simulink model "simulinkTVModel"  (R2023a)
settings: Solver=ode4  StartTime=0.0  StopTime=10.0  FixedStep=0.001  RelTol=1e-3
values from neighbouring files (symbols this model uses):
  K_att1 = lqr(AA,BA,QA,RA)    [TV_SIM_woCA.m]    (also in controllerParams.m)
  K_att2 = inv(BA'*BA)*BA'*AA    [controllerParams.m]
  K_pos1 = lqr(AP,BP,QP,RP)    [TV_SIM_woCA.m]    (also in controllerParams.m)
  K_pos2 = inv(BP'*BP)*BP'*AP    [controllerParams.m]
  x0 = zeros(12,1)    [TV_SIM_woCA.m]    (also in mpc_control_allocation.m = [0 0 0 0 0 0 0 0 0 0 0 0]'; runThrustVectoringQuadrotorModel.m = [0,0,0,0,0,0,0,0,0.2,0,0,0]')
undefined symbols (not defined in the file or in its folder): controlAllocation, TVequationsOfMotion
settings Model: Creator=Jann-AIMLAB  LastModifiedBy=Jann-AIMLAB
settings OptimizationCC: ReuseModelBlockBuffer=off
settings DebuggingCC: UnderSpecifiedDimensionMsg=warning

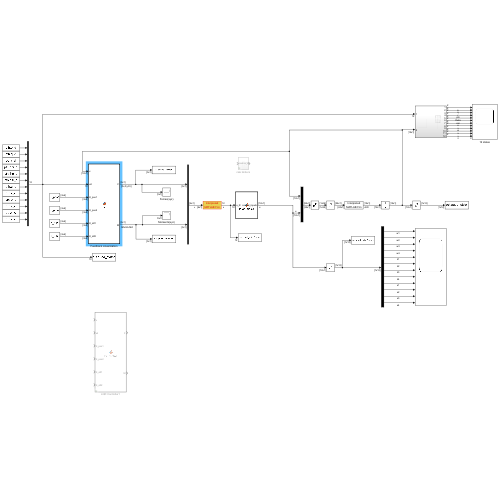
[thumbnail: Simulink's stored preview of the top-level diagram]
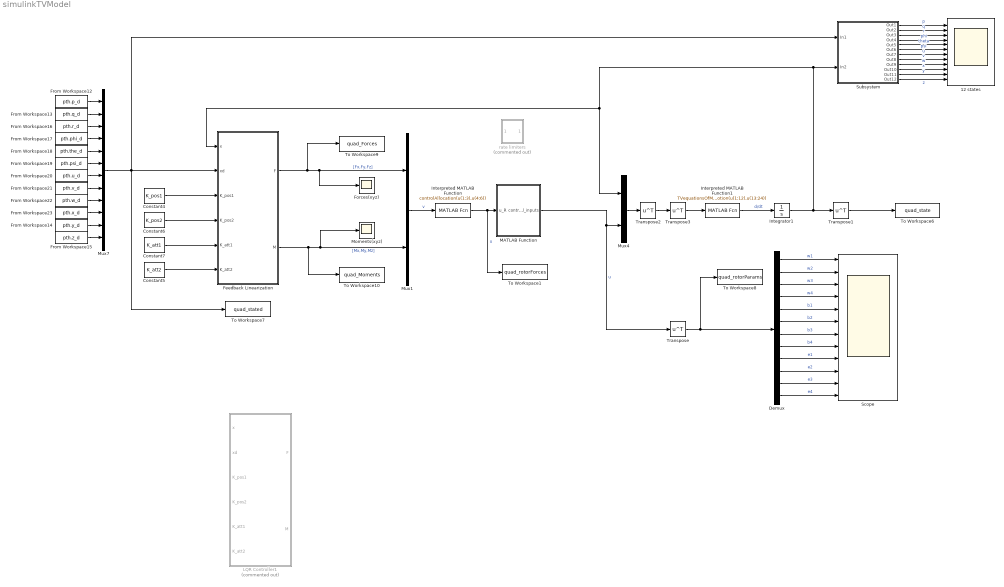
== system simulinkTVModel ==
  12 states : Scope  NumInputPorts=12
  Constant4 : Constant  Value=K_pos1  VectorParams1D=off
  Constant5 : Constant  Value=K_att2  VectorParams1D=off
  Constant6 : Constant  Value=K_pos2  VectorParams1D=off
  Constant7 : Constant  Value=K_att1  VectorParams1D=off
  Demux : Demux  Outputs=12
  Feedback Linearization : MATLAB Function  TreatAsAtomicUnit=on
  Forces(xyz) : Scope
  From Workspace12 : FromWorkspace  VariableName=pth.p_d
  From Workspace13 : FromWorkspace  VariableName=pth.q_d
  From Workspace14 : FromWorkspace  VariableName=pth.y_d
  From Workspace15 : FromWorkspace  VariableName=pth.z_d
  From Workspace16 : FromWorkspace  VariableName=pth.r_d
  From Workspace17 : FromWorkspace  VariableName=pth.phi_d
  From Workspace18 : FromWorkspace  VariableName=pth.the_d
  From Workspace19 : FromWorkspace  VariableName=pth.psi_d
  From Workspace20 : FromWorkspace  VariableName=pth.u_d
  From Workspace21 : FromWorkspace  VariableName=pth.v_d
  From Workspace22 : FromWorkspace  VariableName=pth.w_d
  From Workspace23 : FromWorkspace  VariableName=pth.x_d
  Integrator1 : Integrator  InitialCondition=x0
  Interpreted MATLAB Function : MATLABFcn  MATLABFcn=controlAllocation(u(1:3),u(4:6))
  Interpreted MATLAB Function1 : MATLABFcn  MATLABFcn=TVequationsOfMotion(u(1:12),u(13:24))  Output1D=off
  LQR Controller1 : MATLAB Function  Commented=on  TreatAsAtomicUnit=on
  MATLAB Function : MATLAB Function  TreatAsAtomicUnit=on
  Moments(xyz) : Scope
  Mux1 : Mux  Inputs=2
  Mux4 : Mux  Inputs=2
  Mux7 : Mux  Inputs=12
  Scope : Scope  NumInputPorts=12
  Subsystem : Subsystem
  To Workspace1 : ToWorkspace  VariableName=quad_rotorForces  SampleTime=-1
      settings: Save2DSignal=2-D array (concatenate along first dimension)
  To Workspace10 : ToWorkspace  VariableName=quad_Moments  SaveFormat=Timeseries  SampleTime=-1
  To Workspace6 : ToWorkspace  VariableName=quad_state  SampleTime=-1
      settings: Save2DSignal=2-D array (concatenate along first dimension)
  To Workspace7 : ToWorkspace  VariableName=quad_stated  SaveFormat=Timeseries  SampleTime=-1
  To Workspace8 : ToWorkspace  VariableName=quad_rotorParams  SampleTime=-1
      settings: Save2DSignal=2-D array (concatenate along first dimension)
  To Workspace9 : ToWorkspace  VariableName=quad_Forces  SaveFormat=Timeseries  SampleTime=-1
  Transpose{,1..3} (4 alike) : Math  Operator=transpose
  rate limiters : Subsystem  Commented=on
  wires:
  Subsystem/3(Out3) -> 12 states/3  "r"
  Transpose1/1 -> To Workspace6/1
  Constant6/1 -> Feedback Linearization/4(K_pos2)
  Subsystem/7(Out7) -> 12 states/7  "u"
  From Workspace20/1 -> Mux7/7
  From Workspace16/1 -> Mux7/3
  From Workspace13/1 -> Mux7/2
  Subsystem/11(Out11) -> 12 states/11  "y"
  Subsystem/9(Out9) -> 12 states/9  "w"
  Feedback Linearization/1(F) -> To Workspace9/1, Mux1/1, Forces(xyz)/1  "[Fx,Fy,Fz]"
  Subsystem/6(Out6) -> 12 states/6  "psi"
  Mux4/1 -> Transpose2/1
  Subsystem/10(Out10) -> 12 states/10  "x"
  Interpreted MATLAB Function1/1 -> Integrator1/1  "d/dt"
  From Workspace19/1 -> Mux7/6
  From Workspace23/1 -> Mux7/10
  Subsystem/4(Out4) -> 12 states/4  "phi"
  Mux7/1 -> Subsystem/1(In1), Feedback Linearization/2(xd), To Workspace7/1
  Constant7/1 -> Feedback Linearization/5(K_att1)
  Subsystem/8(Out8) -> 12 states/8  "v"
  From Workspace14/1 -> Mux7/11
  From Workspace12/1 -> Mux7/1
  Constant5/1 -> Feedback Linearization/6(K_att2)
  Subsystem/5(Out5) -> 12 states/5  "theta"
  Feedback Linearization/2(M) -> To Workspace10/1, Mux1/2, Moments(xyz)/1  "[Mx,My,Mz]"
  Constant4/1 -> Feedback Linearization/3(K_pos1)
  From Workspace17/1 -> Mux7/4
  Integrator1/1 -> Subsystem/2(In2), Feedback Linearization/1(x), Mux4/1, Transpose1/1
  From Workspace18/1 -> Mux7/5
  From Workspace21/1 -> Mux7/8
  Subsystem/1(Out1) -> 12 states/1  "p"
  Subsystem/2(Out2) -> 12 states/2  "q"
  From Workspace22/1 -> Mux7/9
  From Workspace15/1 -> Mux7/12
  Subsystem/12(Out12) -> 12 states/12  "z"
  Mux1/1 -> Interpreted MATLAB Function/1  "v"
  Transpose2/1 -> Transpose3/1
  Transpose3/1 -> Interpreted MATLAB Function1/1
  Demux/1 -> Scope/1  "w1"
  Demux/2 -> Scope/2  "w2"
  Demux/3 -> Scope/3  "w3"
  Demux/4 -> Scope/4  "w4"
  Demux/5 -> Scope/5  "b1"
  Demux/6 -> Scope/6  "b2"
  Demux/7 -> Scope/7  "b3"
  Demux/8 -> Scope/8  "b4"
  Demux/9 -> Scope/9  "e1"
  Demux/10 -> Scope/10  "e2"
  Demux/11 -> Scope/11  "e3"
  Demux/12 -> Scope/12  "e4"
  Transpose/1 -> Demux/1, To Workspace8/1
  Interpreted MATLAB Function/1 -> To Workspace1/1, MATLAB Function/1(u_R)  "u"
  MATLAB Function/1(control_inputs) -> Transpose/1, Mux4/2  "u"

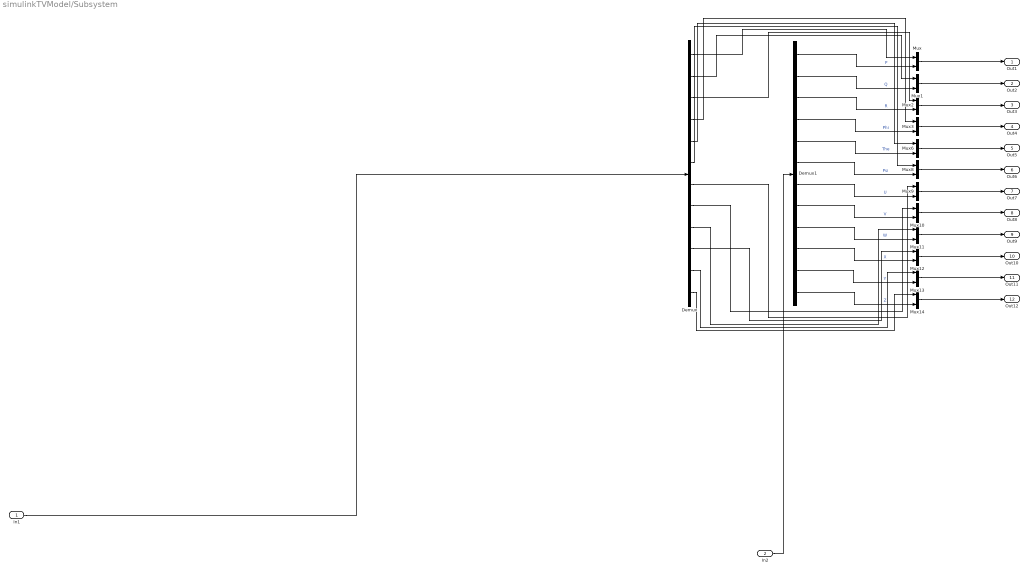
== system simulinkTVModel/Subsystem ==
  In1 : Inport
  In2 : Inport  Port=2
  Demux : Demux  Outputs=12
  Demux1 : Demux  Outputs=12
  Mux{,1..3,6,8..14} (12 alike) : Mux  Inputs=2
  Out1 : Outport
  Out2 : Outport  Port=2
  Out3 : Outport  Port=3
  Out4 : Outport  Port=4
  Out5 : Outport  Port=5
  Out6 : Outport  Port=6
  Out7 : Outport  Port=7
  Out8 : Outport  Port=8
  Out9 : Outport  Port=9
  Out10 : Outport  Port=10
  Out11 : Outport  Port=11
  Out12 : Outport  Port=12
  wires:
  Demux/9 -> Mux11/1
  Demux1/9 -> Mux11/2  "W"
  Demux/7 -> Mux9/1
  In2/1 -> Demux1/1
  Demux1/5 -> Mux6/2  "The"
  Demux1/10 -> Mux12/2  "X"
  Demux1/2 -> Mux1/2  "Q"
  Demux1/7 -> Mux9/2  "U"
  Mux10/1 -> Out8/1
  Demux1/11 -> Mux13/2  "Y"
  Demux/3 -> Mux2/1
  Demux/11 -> Mux13/1
  Demux1/8 -> Mux10/2  "V"
  Mux2/1 -> Out3/1
  Demux/6 -> Mux8/1
  Demux1/4 -> Mux3/2  "Phi"
  Demux/5 -> Mux6/1
  Demux/8 -> Mux10/1
  Demux1/1 -> Mux/2  "P"
  Demux/10 -> Mux12/1
  Mux8/1 -> Out6/1
  Demux1/3 -> Mux2/2  "R"
  Demux/1 -> Mux/1
  Demux1/6 -> Mux8/2  "Psi"
  Mux11/1 -> Out9/1
  Demux1/12 -> Mux14/2  "Z"
  Mux6/1 -> Out5/1
  Mux/1 -> Out1/1
  Demux/12 -> Mux14/1
  Demux/2 -> Mux1/1
  Mux12/1 -> Out10/1
  Demux/4 -> Mux3/1
  Mux13/1 -> Out11/1
  Mux3/1 -> Out4/1
  In1/1 -> Demux/1
  Mux14/1 -> Out12/1
  Mux9/1 -> Out7/1
  Mux1/1 -> Out2/1

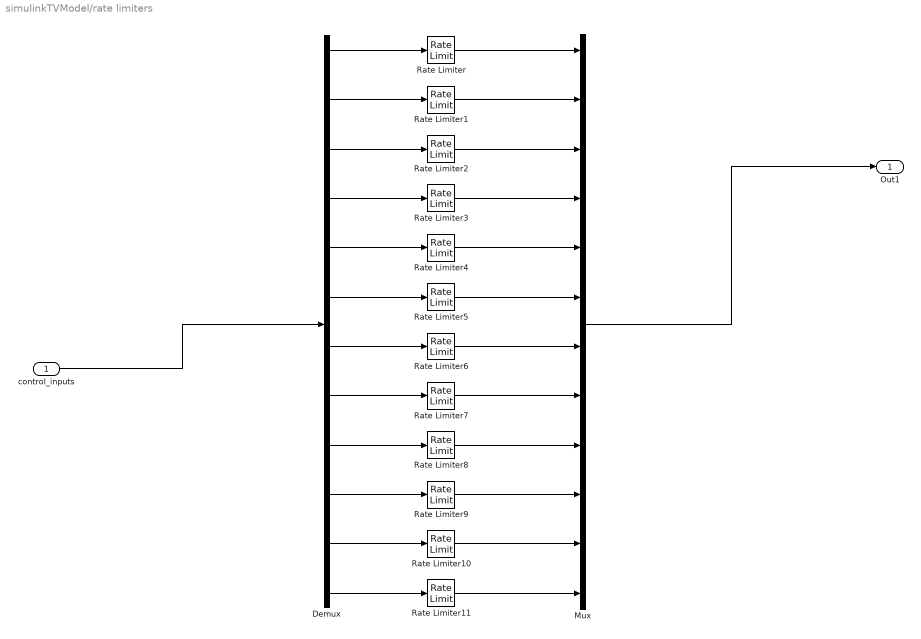
== system simulinkTVModel/rate limiters ==
  control_inputs : Inport
  Demux : Demux  Outputs=12
  Mux : Mux  Inputs=12
  Rate Limiter{,1..3} (4 alike) : RateLimiter  RisingSlewLimit=10000  FallingSlewLimit=-10000  SampleTimeMode=inherited
  Rate Limiter{4..11} (8 alike) : RateLimiter  RisingSlewLimit=100  FallingSlewLimit=-100  SampleTimeMode=inherited
  Out1 : Outport
  wires:
  Demux/1 -> Rate Limiter/1
  Demux/2 -> Rate Limiter1/1
  Demux/3 -> Rate Limiter2/1
  Demux/4 -> Rate Limiter3/1
  control_inputs/1 -> Demux/1
  Demux/5 -> Rate Limiter4/1
  Demux/6 -> Rate Limiter5/1
  Demux/7 -> Rate Limiter6/1
  Demux/8 -> Rate Limiter7/1
  Demux/9 -> Rate Limiter8/1
  Demux/10 -> Rate Limiter9/1
  Demux/11 -> Rate Limiter10/1
  Demux/12 -> Rate Limiter11/1
  Rate Limiter/1 -> Mux/1
  Rate Limiter1/1 -> Mux/2
  Rate Limiter2/1 -> Mux/3
  Rate Limiter3/1 -> Mux/4
  Rate Limiter4/1 -> Mux/5
  Rate Limiter5/1 -> Mux/6
  Rate Limiter6/1 -> Mux/7
  Rate Limiter7/1 -> Mux/8
  Rate Limiter8/1 -> Mux/9
  Rate Limiter9/1 -> Mux/10
  Rate Limiter10/1 -> Mux/11
  Rate Limiter11/1 -> Mux/12
  Mux/1 -> Out1/1

== matlab function simulinkTVModel/LQR Controller1 ==
  data: x input; F output; xd input; K_pos1 input; M output; K_pos2 input; K_att1 input; K_att2 input
function [F,M] = lqr_control(x,xd,K_pos1,K_pos2,K_att1,K_att2)

%states 
%Position       
X = x(10);Y = x(11);Z = x(12);
Xd = xd(10);Yd = xd(11);Zd = xd(12);
%Velocity
U = x(7);V = x(8);W = x(9);
Ud = xd(7);Vd = xd(8);Wd = xd(9);
%Euler Angles
Phi = x(4);The = x(5);Psi = x(6);
Phid = xd(4);Thed = xd(5);Psid = xd(6);
%Body Rates
P = x(1);Q = x(2);R = x(3);
Pd = xd(1);Qd = xd(2);Rd = xd(3);


%position control 
%pos_d = [0;0;0;0;0;0];
pos_d = [Xd;Yd;Zd;Ud;Vd;Wd];
pos = [X;Y;Z;U;V;W];
pos_err = pos_d - pos;
%pos_err = pos - pos_d;

%F = -K_pos1*pos_err;
%F = -K_pos1*pos_err + K_pos2*pos_d; % works as a regulator
F = K_pos1*pos_err + K_pos2*pos_d;



%attitude control
%att_d = [0;0;0;0;0;0];
att_d = [Phid;Thed;Psid;Pd;Qd;Rd];
att = [Phi;The;Psi;P;Q;R];
att_err = att_d-att;
%att_err = att-att_d;
%M = -K_att1*att_err;
%M = K_att1*att_err - K_att2*att_d;
M = K_att1*att_err + K_att2*att_d;



%y = [F(1),F(2),F(3),M(1),M(2),M(3)];

== matlab function simulinkTVModel/MATLAB Function ==
  data: u_R input; control_inputs output
function control_inputs = rotorParams(u_R)

L = [0.225, 0.225, 0];
kT = 2.98e-6;
kQ = 1.140e-7;

e1 = asin((u_R(1))/(sqrt(u_R(1)^2+u_R(2)^2+u_R(3)^2)));
e2 = asin((u_R(4))/(sqrt(u_R(4)^2+u_R(5)^2+u_R(6)^2)));
e3 = -asin((u_R(7))/(sqrt(u_R(7)^2+u_R(8)^2+u_R(9)^2)));
e4 = -asin((u_R(10))/(sqrt(u_R(10)^2+u_R(11)^2+u_R(12)^2)));

b1 = -asin((u_R(2))/(cos(e1)*sqrt(u_R(1)^2+u_R(2)^2+u_R(3)^2)));
b2 = -asin((u_R(5))/(cos(e2)*sqrt(u_R(4)^2+u_R(5)^2+u_R(6)^2)));
b3 = asin((u_R(8))/(cos(e3)*sqrt(u_R(7)^2+u_R(8)^2+u_R(9)^2)));
b4 = asin((u_R(11))/(cos(e4)*sqrt(u_R(10)^2+u_R(11)^2+u_R(12)^2)));

w1 = (30/pi)*sqrt(sqrt(u_R(1)^2+u_R(2)^2+u_R(3)^2)/(kT));
w2 = (30/pi)*sqrt(sqrt(u_R(4)^2+u_R(5)^2+u_R(6)^2)/(kT));
w3 = (30/pi)*sqrt(sqrt(u_R(7)^2+u_R(8)^2+u_R(9)^2)/(kT));
w4 = (30/pi)*sqrt(sqrt(u_R(10)^2+u_R(11)^2+u_R(12)^2)/(kT));

rotorSpeed = [w1,w2,w3,w4];
rotorRoll = [b1,b2,b3,b4];
rotorPitch = [e1,e2,e3,e4];

control_inputs = [w1,w2,w3,w4,b1,b2,b3,b4,e1,e2,e3,e4]';

== matlab function simulinkTVModel/Feedback Linearization ==
  data: x input; F output; xd input; K_pos1 input; M output; K_pos2 input; K_att1 input; K_att2 input
function [F,M] = fbl(x,xd,K_pos1,K_pos2,K_att1,K_att2)
% CALCULATE MOMENT AND THRUST FORCES
%find k,d,l
k=2.98e-06; kQ = 1.14e-7;%kQ=.0382; 
%find m,Ixx,Iyy,Izz,Ir
m=0.468; 
%m = 0.68;
g = 9.81;
Ixx=4.856e-03;Iyy=4.856e-03;Izz=8.801e-03;

Ir=3.357e-05;
Ax=.3; Ay=0.3; Az=0.25; Ar=0.2;

Omega =0;

%Omega = w(1)-w(2)+w(3)-w(4);   
% if size(w) == [1,1]
% Omega = 0;
% else
% Omega = w(1)-w(2)+w(3)-w(4);
% end


% states: x = [p,q,r,phi,the,psi,u,v,w,x,y,z];

% position control
% state error 
e_p = x(7:12) - xd(7:12);
% f_p = -(1/m)*[Ax,0,0,0,0,0;
%                0,Ay,0,0,0,0;
%                0,0,Az + g,0,0,0;
%                1,0,0,0,0,0;
%                0,1,0,0,0,0;
%                0,0,1,0,0,0];
f_p = [-(1/m)*(Ax*x(7));
    -(1/m)*(Ay*x(8));
    -(1/m)*(Az*x(9));
    x(7);
    x(8);
    x(9)];
g_p = (1/m)*[cos(x(6))*cos(x(5)), cos(x(4))*sin(x(6)) + cos(x(6))*sin(x(4))*sin(x(5)), sin(x(4))*sin(x(6)) - cos(x(4))*cos(x(6))*sin(x(5)), 0, 0, 0;
					-cos(x(5))*sin(x(6)), cos(x(4))*cos(x(6)) - sin(x(4))*sin(x(6))*sin(x(5)), cos(x(6))*sin(x(4)) + cos(x(4))*sin(x(6))*sin(x(5)), 0, 0, 0;
					sin(x(5)), -cos(x(5))*sin(x(4)), cos(x(4))*cos(x(5)), 0, 0, 0;
					0,0,0,0,0,0;
					0,0,0,0,0,0;
					0,0,0,0,0,0];

% F = g_p(1:3,1:3)\(-(f_p(4:6).'*f_p(1:3))-10.*K_pos1*e_p-0.*K_pos2*xd(7:12));
%F = m.*(-(f_p(4:6).'*f_p(1:3))-K_pos1*e_p-K_pos2*xd(7:12));
F = g_p(1:3,1:3)\(-(f_p(4:6).'*f_p(1:3))-K_pos1*e_p);

% attitude control 
e_a = x(1:6) - xd(1:6);
f_a = [(1/Ixx)*((Iyy-Izz)*x(2)*x(3)-Ir*x(2)*Omega-Ar*x(1));
    (1/Iyy)*((Ixx-Izz)*x(1)*x(3)-Ir*x(1)*Omega-Ar*x(2));
    (1/Izz)*((Iyy-Ixx)*x(2)*x(1)-Ar*x(3));
    x(1) + sin(x(4))*tan(x(5))*x(2) + cos(x(4))*tan(x(5))*x(3);
    cos(x(4))*x(2) - sin(x(4))*x(3);
    sin(x(4))/cos(x(5))*x(2) + cos(x(4))/cos(x(5))*x(3)];
g_a = [(1/Ixx),0,0,0,0,0;
    0,(1/Iyy),0,0,0,0;
    0,0,(1/Izz),0,0,0;
    0,0,0,0,0,0;
    0,0,0,0,0,0;
    0,0,0,0,0,0];

%M = g_a(1:3,1:3)\(-(f_a(4:6).'*f_a(1:3))-10.*K_att1*e_a-0.*K_att2*xd(1:6));
M = g_a(1:3,1:3)\(-(f_a(4:6).'*f_a(1:3))-K_att1*e_a);











% %states 
% %Position       
% X = x(10);Y = x(11);Z = x(12);
% Xd = xd(10);Yd = xd(11);Zd = xd(12);
% %Velocity
% U = x(7);V = x(8);W = x(9);
% Ud = xd(7);Vd = xd(8);Wd = xd(9);
% %Euler Angles
% Phi = x(4);The = x(5);Psi = x(6);
% Phid = xd(4);Thed = xd(5);Psid = xd(6);
% %Body Rates
% P = x(1);Q = x(2);R = x(3);
% Pd = xd(1);Qd = xd(2);Rd = xd(3);
% 
% 
% %position control 
% %pos_d = [0;0;0;0;0;0];
% pos_d = [Xd;Yd;Zd;Ud;Vd;Wd];
% pos = [X;Y;Z;U;V;W];
% pos_err = pos_d - pos;
% %pos_err = pos - pos_d;
% 
% %F = -K_pos1*pos_err;
% %F = -K_pos1*pos_err + K_pos2*pos_d; % works as a regulator
% F = K_pos1*pos_err + K_pos2*pos_d;
% 
% 
% 
% %attitude control
% %att_d = [0;0;0;0;0;0];
% att_d = [Phid;Thed;Psid;Pd;Qd;Rd];
% att = [Phi;The;Psi;P;Q;R];
% att_err = att_d-att;
% %att_err = att-att_d;
% %M = -K_att1*att_err;
% %M = K_att1*att_err - K_att2*att_d;
% M = K_att1*att_err + K_att2*att_d;



%y = [F(1),F(2),F(3),M(1),M(2),M(3)];
